simulink model "Uklad_simulink_vivado"  (R2025b)
settings: Solver=FixedStepDiscrete  StartTime=0.0  StopTime=20  RelTol=1e-3
undefined symbols (not defined in the file or in its folder): c, sfvc784, xck26
libraries: hdlUtilities x2, hdlDSPIP x1, vmcUtilities x1
settings Model: Creator=janek  LastModifiedBy=janek

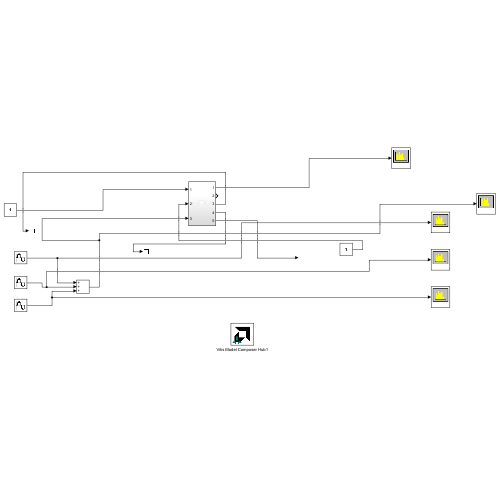
[thumbnail: Simulink's stored preview of the top-level diagram]
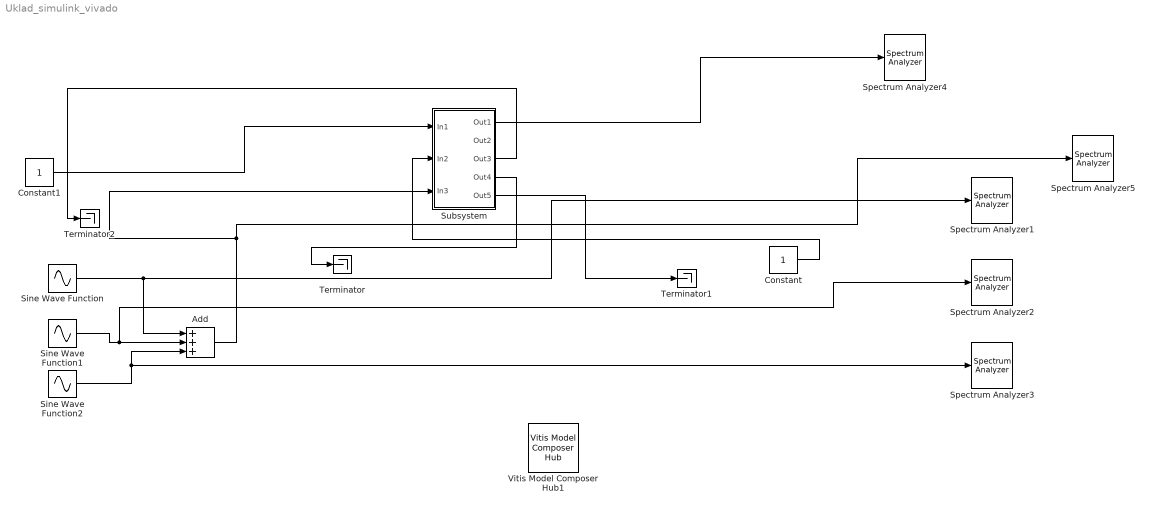
== system Uklad_simulink_vivado ==
  Add : Sum  Inputs=+++
  Constant : Constant  OutDataTypeStr=boolean
  Constant1 : Constant  OutDataTypeStr=boolean
  Sine Wave Function : Sin  Frequency=2*pi*1000  SampleTime=1/27000
  Sine Wave Function1 : Sin  Frequency=2*pi*3500  SampleTime=1/27000
  Sine Wave Function2 : Sin  Frequency=2*pi*7000  SampleTime=1/27000
  Spectrum Analyzer1 : SpectrumAnalyzer  WindowPosition=[2776.000000,2394.000000,1105.000000,500.000000,]  Visible=on  ScopeFrameLocation=window  WindowInvariantSamplesPerUpdate=on  Span=27000  StartFrequency=-13500  StopFrequency=13500  MaximizeAxes=Off  YLimits=[-394.5855396148054 151.1136443372478]
  Spectrum Analyzer2 : SpectrumAnalyzer  WindowPosition=[2772.000000,1814.000000,1105.000000,500.000000,]  Visible=on  ScopeFrameLocation=window  WindowInvariantSamplesPerUpdate=on  Span=27000  StartFrequency=-13500  StopFrequency=13500  YLimits=[-1102.9956638291546 573.1047111409932]
  Spectrum Analyzer3 : SpectrumAnalyzer  WindowPosition=[2752.000000,1245.000000,1105.000000,500.000000,]  Visible=on  ScopeFrameLocation=window  WindowInvariantSamplesPerUpdate=on  Span=27000  StartFrequency=-13500  StopFrequency=13500  YLimits=[-2154.3264776502465 1159.3055172489956]
  Spectrum Analyzer4 : SpectrumAnalyzer  WindowPosition=[2776.000000,2981.000000,1105.000000,500.000000,]  Visible=on  ScopeFrameLocation=window  WindowInvariantSamplesPerUpdate=on  Span=27000  StartFrequency=-13500  StopFrequency=13500  YLimits=[-251.3612 53.9685]
  Spectrum Analyzer5 : SpectrumAnalyzer  WindowPosition=[-1290.000000,2968.000000,1105.000000,500.000000,]  Visible=on  ScopeFrameLocation=window  WindowInvariantSamplesPerUpdate=on  Span=27000  StartFrequency=-13500  StopFrequency=13500  YLimits=[-245.3447 53.9043]
  Subsystem : Subsystem
  Terminator : Terminator
  Terminator1 : Terminator
  Terminator2 : Terminator
  Vitis Model Composer Hub1 : vmcUtilities/Vitis Model Composer Hub  Tag=genX  CodeGeneration=off  SubsystemName=Subsystem  CompilationType=HDLCompilation  ExportTypeV2=IP Catalog  StartColumn=1  NumberOfColumns=1  TargetDirectory=./netlist  exportDesign=off  analyzeDesign=off  validateDesignOnHw=off  ExportType=AI Engines  IpVendor=xilinx.com  IpLibrary=hls  IpVersion=1.0  IpHWLanguage=Verilog  AieCompilerOptions={}  AieSimulatorOptions={}  CreateTestbench=off  TestbenchStackSize=10  RunRtlSim=off  RunCSim=off  RunAieSim=off  AieSimTimeout=50000  RunAieSimProfiling=off  LaunchVitisAnalyzer=off  PlotOutput=off  RunX86Sim=off  X86SimTimeout=10  GenHwImage=off  GenLibadfXo=on  GenHwValidationCode=off  PlatformType=Not Specified  HwSystemType=Baremetal  HwValidationTarget=hw  ProjDevice=Kria KR260 Robotics Starter Kit SOM (xck26-sfvc784-2LV-c)  ProjDevicePart=xck26-sfvc784-2LV-c  AIEType=None  SamplePeriod=-1  ClockFrequency=200  DataPathParallelism=1  xilinxfamily=zynquplus  part=xck26  speed=-2LV-c  package=sfvc784  directory=./netlist\ip\Subsystem\src  testbench=off  incr_netlist=off  synthesis_tool=Vivado  clock_wrapper=Clock Enables  dbl_ovrd=According to Block Masks  dcm_input_clock_period=10  sysclk_period=10  simulink_period=1/27000  eval_field=0  LogFileName=''  NThreads=4
  wires:
  Sine Wave Function/1 -> Spectrum Analyzer1/1, Add/1
  Sine Wave Function1/1 -> Spectrum Analyzer2/1, Add/2
  Sine Wave Function2/1 -> Spectrum Analyzer3/1, Add/3
  Constant1/1 -> Subsystem/1(In1)
  Constant/1 -> Subsystem/2(In2)
  Add/1 -> Spectrum Analyzer5/1, Subsystem/3(In3)
  Subsystem/1(Out1) -> Spectrum Analyzer4/1
  Subsystem/3(Out3) -> Terminator2/1
  Subsystem/4(Out4) -> Terminator/1
  Subsystem/5(Out5) -> Terminator1/1

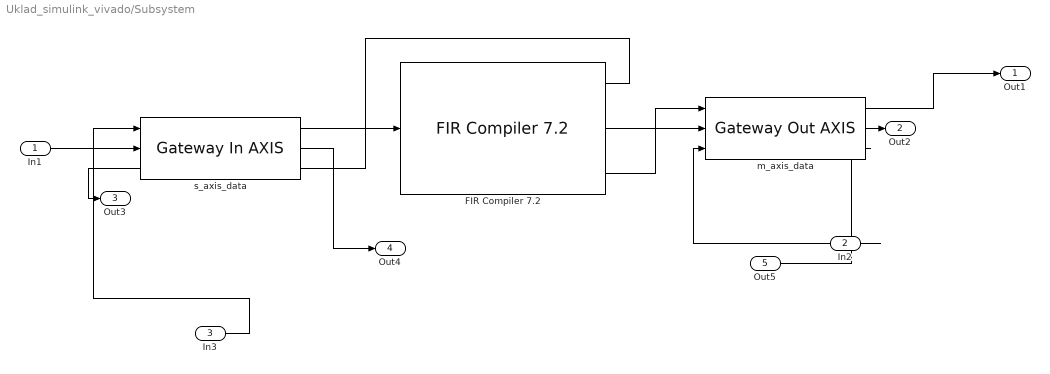
== system Uklad_simulink_vivado/Subsystem ==
  In1 : Inport
  In2 : Inport  Port=2
  In3 : Inport  Port=3
  "FIR Compiler 7.2 " : hdlDSPIP/FIR Compiler 7.2   coefficientvector=my_coefficients  coefficient_sets=1  coefficient_reload=off  filter_type=Single_Rate  rate_change_type=Integer  interpolation_rate=1  decimation_rate=1  zero_pack_factor=1  channel_sequence=Basic  number_channels=1  pattern_list='P4-0,P4-1,P4-2,P4-3,P4-4'  number_paths=1  ratespecification=Maximum_Possible  sampleperiod=1  hardwareoversamplingrate=1  coefficient_sign=Unsigned  quantization=Quantize_Only  coefficient_width=16  bestprecision=on  coefficient_fractional_bits=16  coefficient_structure=Inferred  output_rounding_mode=Full_Precision  output_width=34  filter_architecture=Systolic_Multiply_Accumulate  optimization_goal=Area  optimization_list='None'  data_buffer_type=Automatic  coefficient_buffer_type=Automatic  input_buffer_type=Automatic  output_buffer_type=Automatic  preference_for_other_storage=Automatic  multi_column_support=Automatic  columnconfig='69'  inter_column_pipe_length=4  data_has_tlast=Not_Required  m_data_has_tready=off  s_data_has_fifo=off  s_data_has_tuser=Not_Required  m_data_has_tuser=Not_Required  s_config_sync_mode=On_Vector  s_config_method=Single  num_reload_slots=1  has_aclken=off  has_aresetn=off  reset_data_vector=on  trim_axipin_name=on  simulation_type=hybrid_sim  simulation_model=sysgen:xfirv7_2_cmodel  data_path_portlist={ 's_axis_data_tdata', 'm_axis_data_tdata' }  passband_min=0.0  passband_max=0.5  stopband_min=0.5  stopband_max=1.0  filter_selection=1  gui_behaviour='Sysgen_GUI'  data_sign=Signed  data_width=16  data_fractional_bits=0  data_tuser_width=1  wrapper_available=true  ip_wrap_arbitrary_binary_point=true  ip_name=FIR Compiler  ip_version=7.2  dsptool_ready=true  ipcore_usecache=true  ipcore_useipmodelcache=true  port_translation_map={ 'aclken' => 'en', 'aresetn' => 'rst' }  run_core_at_system_period=true  ipcore_xco_need_fpga_part=true  ipcore_fpga_part=[]  XmcBlockStatus=1  maskContainerNames=tabcontainer1  block_type=fir_compiler_v7_2  block_config=sysgen:rodinimport_config  block_width=820  block_height=600
  m_axis_data : hdlUtilities/Gateway Out AXIS  mask_sample_period=1/27000  bool_to_boolean=off  block_type=gatewayoutaxi
  s_axis_data : hdlUtilities/Gateway In AXIS  gui_display_data_type=Fixed-point  arith_type=Signed (2's comp)  n_bits=16  bin_pt=12  preci_type=Custom  exp_width=16  frac_width=24  quantization="Round  (unbiased: +/- Inf)"  overflow=Saturate  bool_to_boolean=off  OutSampleTime=1/27000  block_type=gatewayinaxi  XmcBlockStatus=1
      link override s_axis_data_tdata: gui_display_data_type=Fixed-point
  Out1 : Outport
  Out2 : Outport  Port=2
  Out3 : Outport  Port=3
  Out4 : Outport  Port=4
  Out5 : Outport  Port=5
  wires:
  s_axis_data/3 -> Out3/1
  m_axis_data/3 -> Out5/1
  In3/1 -> s_axis_data/1
  s_axis_data/1 -> "FIR Compiler 7.2 "/1
  "FIR Compiler 7.2 "/2 -> m_axis_data/2
  m_axis_data/2 -> Out2/1
  In1/1 -> s_axis_data/2
  In2/1 -> m_axis_data/3
  m_axis_data/1 -> Out1/1
  "FIR Compiler 7.2 "/1 -> s_axis_data/3
  "FIR Compiler 7.2 "/3 -> m_axis_data/1
  s_axis_data/2 -> Out4/1
